simulink model "TST_CoEng_Mon"  (R2016b)
settings: Solver=FixedStepDiscrete  StartTime=0.0  StopTime=simTime  FixedStep=sampleTime  RelTol=1e-3
values from neighbouring files (symbols this model uses):
  testCase = 1    [initTST_CoEng_Mon_001.m]
libraries: simulink x3, UnitTest_Lib x1
settings Model: Creator=zhengjinyan  LastModifiedBy=zhengjinyan
settings DebuggingCC: SignalRangeChecking=error

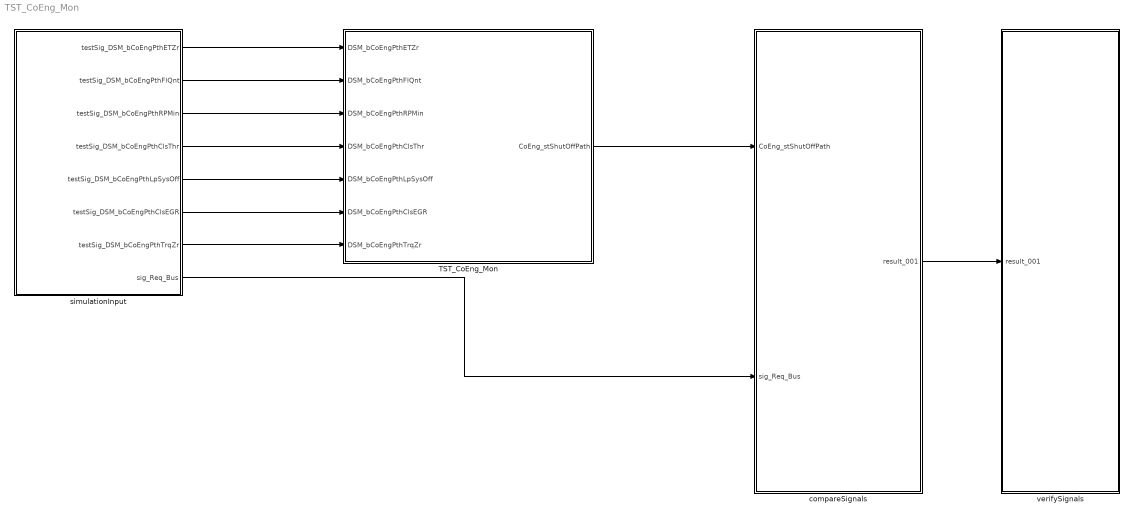
== system TST_CoEng_Mon ==
  TST_CoEng_Mon : Subsystem
  compareSignals : Subsystem
  simulationInput : Subsystem
  verifySignals : Subsystem
  wires:
  simulationInput/1(testSig_DSM_bCoEngPthETZr) -> TST_CoEng_Mon/1(DSM_bCoEngPthETZr)
  simulationInput/2(testSig_DSM_bCoEngPthFlQnt) -> TST_CoEng_Mon/2(DSM_bCoEngPthFlQnt)
  simulationInput/3(testSig_DSM_bCoEngPthRPMin) -> TST_CoEng_Mon/3(DSM_bCoEngPthRPMin)
  simulationInput/4(testSig_DSM_bCoEngPthClsThr) -> TST_CoEng_Mon/4(DSM_bCoEngPthClsThr)
  simulationInput/5(testSig_DSM_bCoEngPthLpSysOff) -> TST_CoEng_Mon/5(DSM_bCoEngPthLpSysOff)
  simulationInput/6(testSig_DSM_bCoEngPthClsEGR) -> TST_CoEng_Mon/6(DSM_bCoEngPthClsEGR)
  simulationInput/7(testSig_DSM_bCoEngPthTrqZr) -> TST_CoEng_Mon/7(DSM_bCoEngPthTrqZr)
  TST_CoEng_Mon/1(CoEng_stShutOffPath) -> compareSignals/1(CoEng_stShutOffPath)
  simulationInput/8(sig_Req_Bus) -> compareSignals/2(sig_Req_Bus)
  compareSignals/1(result_001) -> verifySignals/1(result_001)

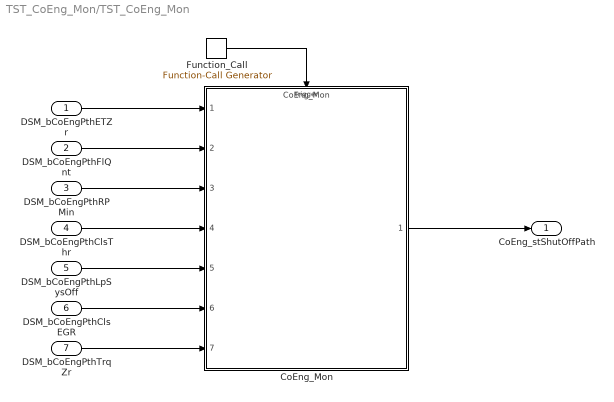
== system TST_CoEng_Mon/TST_CoEng_Mon ==
  DSM_bCoEngPthETZr : Inport
  DSM_bCoEngPthFlQnt : Inport  Port=2
  DSM_bCoEngPthRPMin : Inport  Port=3
  DSM_bCoEngPthClsThr : Inport  Port=4
  DSM_bCoEngPthLpSysOff : Inport  Port=5
  DSM_bCoEngPthClsEGR : Inport  Port=6
  DSM_bCoEngPthTrqZr : Inport  Port=7
  CoEng_Mon : ModelReference  ModelNameDialog=CoEng_Mon  SimulationMode=Normal  ModelReferenceVersion=1.3  TriggerPortName=function  TriggerPortTriggerType=function-call  TriggerPortStatesWhenEnabling=held
  Function_Call : simulink/Ports & Subsystems/Function-Call Generator  sample_time=sampleTime  numberOfIterations=1
  CoEng_stShutOffPath : Outport
  wires:
  Function_Call/1 -> CoEng_Mon/Trigger
  DSM_bCoEngPthETZr/1 -> CoEng_Mon/1
  DSM_bCoEngPthFlQnt/1 -> CoEng_Mon/2
  DSM_bCoEngPthRPMin/1 -> CoEng_Mon/3
  DSM_bCoEngPthClsThr/1 -> CoEng_Mon/4
  DSM_bCoEngPthLpSysOff/1 -> CoEng_Mon/5
  DSM_bCoEngPthClsEGR/1 -> CoEng_Mon/6
  DSM_bCoEngPthTrqZr/1 -> CoEng_Mon/7
  CoEng_Mon/1 -> CoEng_stShutOffPath/1

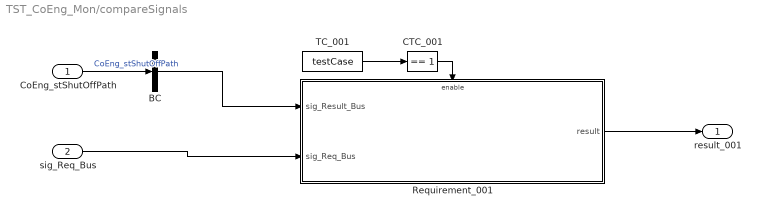
== system TST_CoEng_Mon/compareSignals ==
  CoEng_stShutOffPath : Inport
  sig_Req_Bus : Inport  Port=2
  BC : BusCreator  Inputs=1
  CTC_001 : simulink/Logic and Bit Operations/Compare To Constant  relop===  const=1  OutDataTypeStr=boolean
  Requirement_001 : Subsystem
  TC_001 : Constant  Value=testCase
  result_001 : Outport
  wires:
  CoEng_stShutOffPath/1 -> BC/1  "CoEng_stShutOffPath"
  TC_001/1 -> CTC_001/1
  CTC_001/1 -> Requirement_001/Enable
  sig_Req_Bus/1 -> Requirement_001/2(sig_Req_Bus)
  BC/1 -> Requirement_001/1(sig_Result_Bus)
  Requirement_001/1(result) -> result_001/1

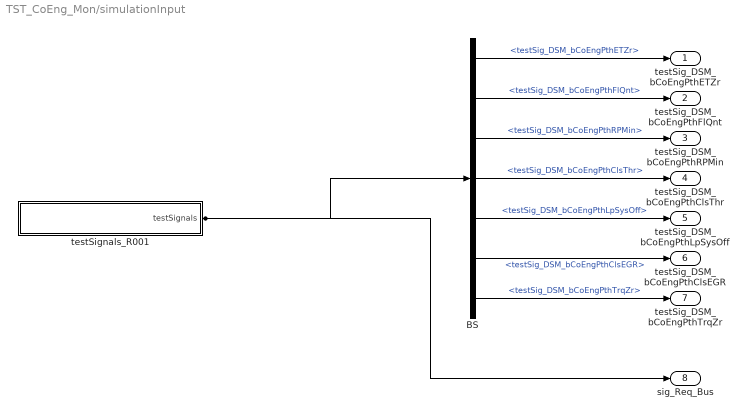
== system TST_CoEng_Mon/simulationInput ==
  BS : BusSelector  OutputSignals=testSig_DSM_bCoEngPthETZr,testSig_DSM_bCoEngPthFlQnt,testSig_DSM_bCoEngPthRPMin,testSig_DSM_bCoEngPthClsThr,testSig_DSM_bCoEngPthLpSysOff,testSig_DSM_bCoEngPthClsEGR,testSig_DSM_bCoEngPthTrqZr
  testSignals_R001 : Subsystem
  testSig_DSM_bCoEngPthETZr : Outport
  testSig_DSM_bCoEngPthFlQnt : Outport  Port=2
  testSig_DSM_bCoEngPthRPMin : Outport  Port=3
  testSig_DSM_bCoEngPthClsThr : Outport  Port=4
  testSig_DSM_bCoEngPthLpSysOff : Outport  Port=5
  testSig_DSM_bCoEngPthClsEGR : Outport  Port=6
  testSig_DSM_bCoEngPthTrqZr : Outport  Port=7
  sig_Req_Bus : Outport  Port=8
  wires:
  BS/1 -> testSig_DSM_bCoEngPthETZr/1  "<testSig_DSM_bCoEngPthETZr>"
  BS/2 -> testSig_DSM_bCoEngPthFlQnt/1  "<testSig_DSM_bCoEngPthFlQnt>"
  BS/3 -> testSig_DSM_bCoEngPthRPMin/1  "<testSig_DSM_bCoEngPthRPMin>"
  BS/4 -> testSig_DSM_bCoEngPthClsThr/1  "<testSig_DSM_bCoEngPthClsThr>"
  BS/5 -> testSig_DSM_bCoEngPthLpSysOff/1  "<testSig_DSM_bCoEngPthLpSysOff>"
  BS/6 -> testSig_DSM_bCoEngPthClsEGR/1  "<testSig_DSM_bCoEngPthClsEGR>"
  BS/7 -> testSig_DSM_bCoEngPthTrqZr/1  "<testSig_DSM_bCoEngPthTrqZr>"
  testSignals_R001/1(testSignals) -> BS/1, sig_Req_Bus/1

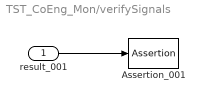
== system TST_CoEng_Mon/verifySignals ==
  result_001 : Inport
  Assertion_001 : Assertion  Enabled=off
  wires:
  result_001/1 -> Assertion_001/1

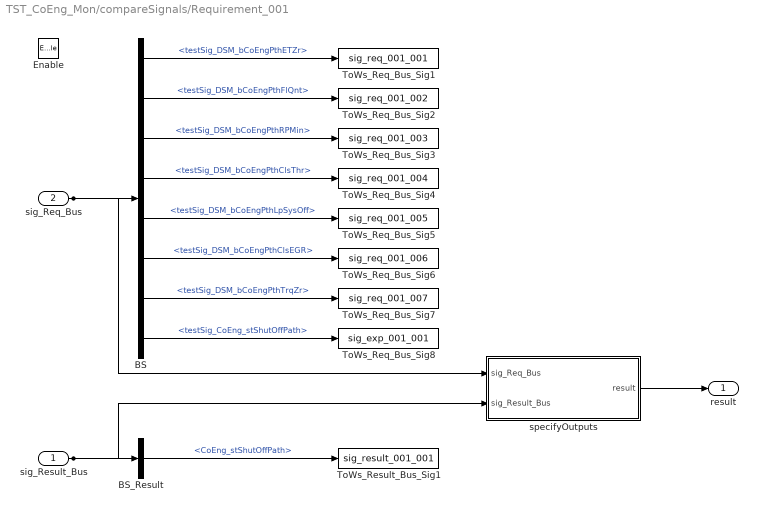
== system TST_CoEng_Mon/compareSignals/Requirement_001 ==
  sig_Result_Bus : Inport
  sig_Req_Bus : Inport  Port=2
  Enable : EnablePort
  BS : BusSelector  OutputSignals=testSig_DSM_bCoEngPthETZr,testSig_DSM_bCoEngPthFlQnt,testSig_DSM_bCoEngPthRPMin,testSig_DSM_bCoEngPthClsThr,testSig_DSM_bCoEngPthLpSysOff,testSig_DSM_bCoEngPthClsEGR,testSig_DSM_bCoEngPthTrqZr,testSig_CoEng_stShutOffPath
  BS_Result : BusSelector  OutputSignals=CoEng_stShutOffPath
  ToWs_Req_Bus_Sig1 : ToWorkspace  VariableName=sig_req_001_001  SaveFormat=Structure With Time
  ToWs_Req_Bus_Sig2 : ToWorkspace  VariableName=sig_req_001_002  SaveFormat=Structure With Time
  ToWs_Req_Bus_Sig3 : ToWorkspace  VariableName=sig_req_001_003  SaveFormat=Structure With Time
  ToWs_Req_Bus_Sig4 : ToWorkspace  VariableName=sig_req_001_004  SaveFormat=Structure With Time
  ToWs_Req_Bus_Sig5 : ToWorkspace  VariableName=sig_req_001_005  SaveFormat=Structure With Time
  ToWs_Req_Bus_Sig6 : ToWorkspace  VariableName=sig_req_001_006  SaveFormat=Structure With Time
  ToWs_Req_Bus_Sig7 : ToWorkspace  VariableName=sig_req_001_007  SaveFormat=Structure With Time
  ToWs_Req_Bus_Sig8 : ToWorkspace  VariableName=sig_exp_001_001  SaveFormat=Structure With Time
  ToWs_Result_Bus_Sig1 : ToWorkspace  VariableName=sig_result_001_001  SaveFormat=Structure With Time
  specifyOutputs : Subsystem
  result : Outport
  wires:
  sig_Req_Bus/1 -> BS/1, specifyOutputs/1(sig_Req_Bus)
  BS/1 -> ToWs_Req_Bus_Sig1/1  "<testSig_DSM_bCoEngPthETZr>"
  BS/2 -> ToWs_Req_Bus_Sig2/1  "<testSig_DSM_bCoEngPthFlQnt>"
  BS/3 -> ToWs_Req_Bus_Sig3/1  "<testSig_DSM_bCoEngPthRPMin>"
  BS/4 -> ToWs_Req_Bus_Sig4/1  "<testSig_DSM_bCoEngPthClsThr>"
  BS/5 -> ToWs_Req_Bus_Sig5/1  "<testSig_DSM_bCoEngPthLpSysOff>"
  BS/6 -> ToWs_Req_Bus_Sig6/1  "<testSig_DSM_bCoEngPthClsEGR>"
  BS/7 -> ToWs_Req_Bus_Sig7/1  "<testSig_DSM_bCoEngPthTrqZr>"
  BS/8 -> ToWs_Req_Bus_Sig8/1  "<testSig_CoEng_stShutOffPath>"
  sig_Result_Bus/1 -> BS_Result/1, specifyOutputs/2(sig_Result_Bus)
  BS_Result/1 -> ToWs_Result_Bus_Sig1/1  "<CoEng_stShutOffPath>"
  specifyOutputs/1(result) -> result/1

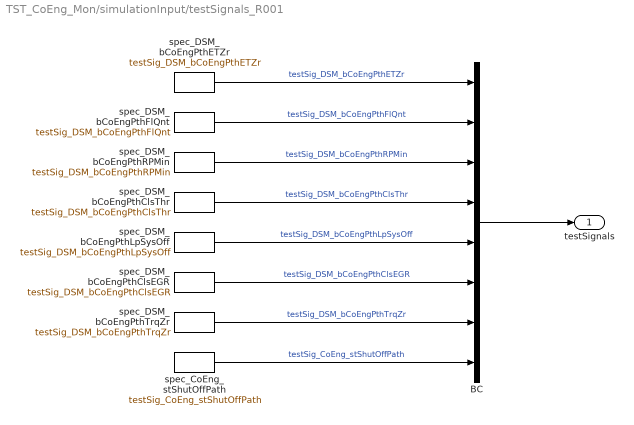
== system TST_CoEng_Mon/simulationInput/testSignals_R001 ==
  BC : BusCreator  Inputs=8
  spec_CoEng_stShutOffPath : FromWorkspace  VariableName=testSig_CoEng_stShutOffPath  Interpolate=off  OutputAfterFinalValue=Holding final value
  spec_DSM_bCoEngPthClsEGR : FromWorkspace  VariableName=testSig_DSM_bCoEngPthClsEGR  Interpolate=off  OutputAfterFinalValue=Holding final value
  spec_DSM_bCoEngPthClsThr : FromWorkspace  VariableName=testSig_DSM_bCoEngPthClsThr  Interpolate=off  OutputAfterFinalValue=Holding final value
  spec_DSM_bCoEngPthETZr : FromWorkspace  VariableName=testSig_DSM_bCoEngPthETZr  Interpolate=off  OutputAfterFinalValue=Holding final value
  spec_DSM_bCoEngPthFlQnt : FromWorkspace  VariableName=testSig_DSM_bCoEngPthFlQnt  Interpolate=off  OutputAfterFinalValue=Holding final value
  spec_DSM_bCoEngPthLpSysOff : FromWorkspace  VariableName=testSig_DSM_bCoEngPthLpSysOff  Interpolate=off  OutputAfterFinalValue=Holding final value
  spec_DSM_bCoEngPthRPMin : FromWorkspace  VariableName=testSig_DSM_bCoEngPthRPMin  Interpolate=off  OutputAfterFinalValue=Holding final value
  spec_DSM_bCoEngPthTrqZr : FromWorkspace  VariableName=testSig_DSM_bCoEngPthTrqZr  Interpolate=off  OutputAfterFinalValue=Holding final value
  testSignals : Outport
  wires:
  BC/1 -> testSignals/1
  spec_DSM_bCoEngPthETZr/1 -> BC/1  "testSig_DSM_bCoEngPthETZr"
  spec_DSM_bCoEngPthFlQnt/1 -> BC/2  "testSig_DSM_bCoEngPthFlQnt"
  spec_DSM_bCoEngPthRPMin/1 -> BC/3  "testSig_DSM_bCoEngPthRPMin"
  spec_DSM_bCoEngPthClsThr/1 -> BC/4  "testSig_DSM_bCoEngPthClsThr"
  spec_DSM_bCoEngPthLpSysOff/1 -> BC/5  "testSig_DSM_bCoEngPthLpSysOff"
  spec_DSM_bCoEngPthClsEGR/1 -> BC/6  "testSig_DSM_bCoEngPthClsEGR"
  spec_DSM_bCoEngPthTrqZr/1 -> BC/7  "testSig_DSM_bCoEngPthTrqZr"
  spec_CoEng_stShutOffPath/1 -> BC/8  "testSig_CoEng_stShutOffPath"

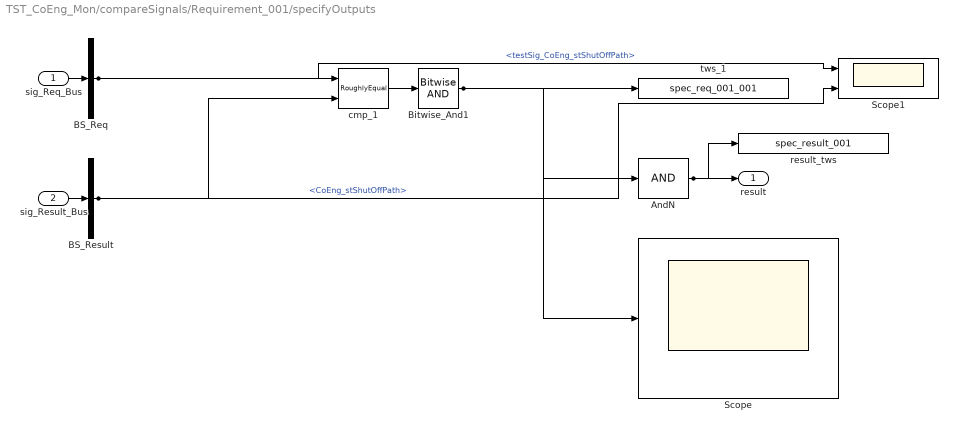
== system TST_CoEng_Mon/compareSignals/Requirement_001/specifyOutputs ==
  sig_Req_Bus : Inport
  sig_Result_Bus : Inport  Port=2
  AndN : Logic  Inputs=1
  BS_Req : BusSelector  OutputSignals=testSig_CoEng_stShutOffPath
  BS_Result : BusSelector  OutputSignals=CoEng_stShutOffPath
  Bitwise_And1 : simulink/Logic and Bit Operations/Bitwise Operator  logicop=AND  UseBitMask=off  BitMask=bin2dec('11011001')  BitMaskRealWorld=Stored Integer
  Scope : Scope
  Scope1 : Scope  NumInputPorts=2
  cmp_1 : UnitTest_Lib/RoughlyEqual  slope=0.1
  result_tws : ToWorkspace  VariableName=spec_result_001
  tws_1 : ToWorkspace  VariableName=spec_req_001_001
  result : Outport
  wires:
  sig_Req_Bus/1 -> BS_Req/1
  sig_Result_Bus/1 -> BS_Result/1
  AndN/1 -> result/1, result_tws/1
  BS_Req/1 -> cmp_1/1, Scope1/1  "<testSig_CoEng_stShutOffPath>"
  BS_Result/1 -> cmp_1/2, Scope1/2  "<CoEng_stShutOffPath>"
  cmp_1/1 -> Bitwise_And1/1
  Bitwise_And1/1 -> tws_1/1, AndN/1, Scope/1
